simulink model "Motivedisplay"  (R2016b)
settings: Solver=ode1  StartTime=0.0  StopTime=inf  FixedStep=0.2  RelTol=1e-3  EnableMultiTasking=on
settings Model: ExtModeTrigDuration=5000  Creator=adm-drone  LastModifiedBy=Control Lab
settings SolverCC: PositivePriorityOrder=on
settings DataIOCC: LimitDataPoints=on  SaveFormat=Array
settings OptimizationCC: LifeSpan=inf
settings DebuggingCC: UnderspecifiedInitializationDetection=Classic  MergeDetectMultiDrivingBlocksExec=none  SolverPrmCheckMsg=warning  StateNameClashWarn=warning  SFUnexpectedBacktrackingDiag=warning  SFNoUnconditionalDefaultTransitionDiag=warning  SFExecutionAtInitializationDiag=none
settings HardwareCC: ProdBitPerPointer=32  ProdBitPerSizeT=32  ProdBitPerPtrDiffT=32  ProdLargestAtomicFloat=None  ProdIntDivRoundTo=Undefined  ProdEndianess=Unspecified  ProdWordSize=32  ProdHWDeviceType=32-bit Generic
settings ModelReferenceCC: PropagateSignalLabelsOutOfModel=off
settings RTWCC: SystemTargetFile=quarc_win64.tlc  TemplateMakefile=quarc_default_tmf  Description=QUARC Win64 Target
settings STFCustomTargetCC: TargetPreCompLibLocation=C:\PROGRA~3\QUARC\lib\2013a\win64\release  GeneratePreprocessorConditionals=Disable all  CombineOutputUpdateFcns=on  CPPClassGenCompliant=on  GRTInterface=off  SystemTargetFile=quarc_win64.tlc
settings GRTTargetCC: TargetPreCompLibLocation=C:\PROGRA~3\QUARC\lib\2013a\win64\release  TargetLangStandard=C89/C90 (ANSI)  ParMdlRefBuildCompliant=off  CompOptLevelCompliant=off  ConcurrentExecutionCompliant=off  GeneratePreprocessorConditionals=Disable all  MatFileLogging=off  UseToolchainInfoCompliant=off  ExtMode=on  ExtModeMexFile=quarc_comm
settings ConfigComp: CovMetricSettings=dw  CovHtmlReporting=on  CovSaveCumulativeToWorkspaceVar=on  CovSaveSingleToWorkspaceVar=on  CovExternalEMLEnable=off

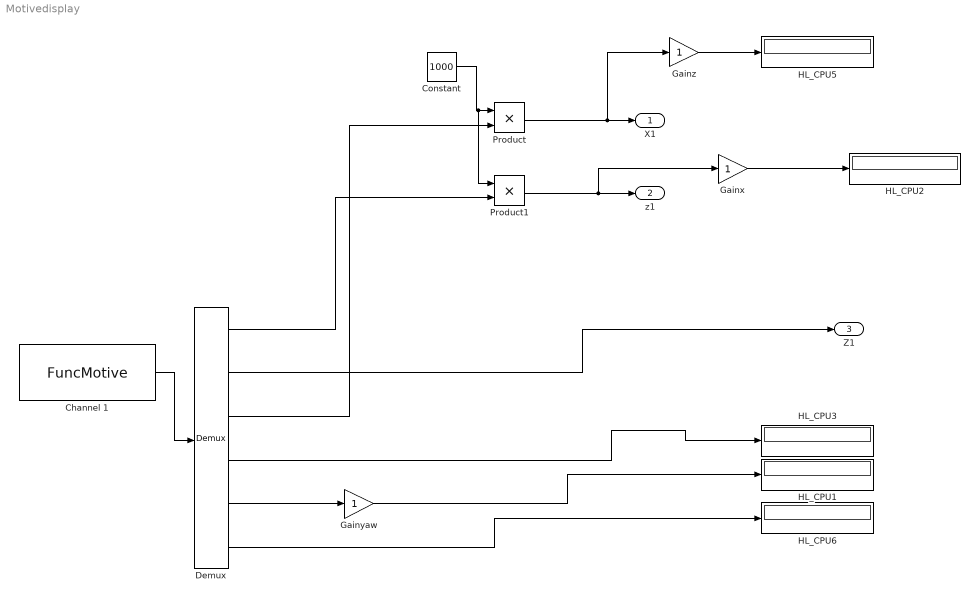
== system Motivedisplay ==
  Channel 1 : M-S-Function  FunctionName=FuncMotive  Parameters=1
  Constant : Constant  Value=1000
  Demux : Demux  Outputs=6
  Gainx : Gain
  Gainyaw : Gain
  Gainz : Gain
  HL_CPU{1..3,5..6} (5 alike) : Display
  Product : Product
  Product1 : Product
  X1 : Outport
  z1 : Outport  Port=2
  Z1 : Outport  Port=3
  wires:
  Channel 1/1 -> Demux/1
  Demux/1 -> Product1/2
  Demux/2 -> Z1/1
  Demux/3 -> Product/2
  Constant/1 -> Product1/1, Product/1
  Product/1 -> Gainz/1, X1/1
  Product1/1 -> Gainx/1, z1/1
  Demux/6 -> HL_CPU6/1
  Demux/4 -> HL_CPU3/1
  Gainz/1 -> HL_CPU5/1
  Gainx/1 -> HL_CPU2/1
  Demux/5 -> Gainyaw/1
  Gainyaw/1 -> HL_CPU1/1
